simulink model "Experiments"  (R2024b)
settings: Solver=ode1  StartTime=0.0  StopTime=30  FixedStep=0.002  RelTol=1e-3  EnableMultiTasking=on
values from neighbouring files (symbols this model uses):
  A = [-2  1  -1  1  0  0 ... (first row only)    [observer_sim.m]    (also in setup_experiments.m = -19.637526957)
  B = eye(n_x,n_u)    [observer_sim.m]    (also in setup_experiments.m = 23*sqrt(4+A^2))
  C = eye(n_y,n_x)    [observer_sim.m]    (also in setup_experiments.m = 1)
  d1_max = 0.8    [observer_sim.m]    (also in setup_experiments.m)
  d1_min = 0.2    [observer_sim.m]    (also in setup_experiments.m)
  epsilon = 0.01    [observer_sim.m]    (also in setup_experiments.m = 0.05)
  L_region1_R = zeros(n_x+n_u, n_y, 2^n_u)    [observer_sim.m]    (also in setup_experiments.m)
  L_region2_R = zeros(n_x+n_u, n_y, 2^n_u)    [observer_sim.m]    (also in setup_experiments.m)
  M = 5    [setup_experiments.m]
  n_u = 2    [observer_sim.m]    (also in setup_experiments.m = 1)
  n_x = 6    [observer_sim.m]    (also in setup_experiments.m = 1)
  n_y = 2    [observer_sim.m]    (also in setup_experiments.m = 1)
  u1dot_max = 10    [observer_sim.m]    (also in setup_experiments.m = 5)
  u1dot_min = -10    [observer_sim.m]    (also in setup_experiments.m = -5)
  w = 1    [setup_experiments.m]
undefined symbols (not defined in the file or in its folder): HIL, qc_get_step_size
libraries: quarc_library x3
settings Model: SimulationMode=external  ExtModeTrigDuration=40000  Creator=MLevis  LastModifiedBy=torivarhaughom
settings SolverCC: AlgebraicLoopSolver=TrustRegion  PositivePriorityOrder=on
settings DataIOCC: SaveFormat=Array  SignalLoggingSaveFormat=ModelDataLogs  ReturnWorkspaceOutputs=off
settings OptimizationCC: ExpressionDepthLimit=2147483647  LifeSpan=inf
settings DebuggingCC: UnderspecifiedInitializationDetection=Classic  MergeDetectMultiDrivingBlocksExec=none  SolverPrmCheckMsg=warning  FcnCallInpInsideContextMsg=warning  UnconnectedInputMsg=warning  UnconnectedOutputMsg=warning  UnconnectedLineMsg=warning  StateNameClashWarn=warning  SFUnexpectedBacktrackingDiag=warning  SFNoUnconditionalDefaultTransitionDiag=warning  SFExecutionAtInitializationDiag=none  ArithmeticOperatorsInVariantConditions=warning
settings HardwareCC: ProdBitPerPointer=32  ProdBitPerSizeT=32  ProdBitPerPtrDiffT=32  ProdLargestAtomicFloat=None  ProdIntDivRoundTo=Undefined  ProdEndianess=Unspecified  ProdWordSize=32  ProdHWDeviceType=32-bit Generic
settings ModelReferenceCC: EnableRefExpFcnMdlSchedulingChecks=on  PropagateSignalLabelsOutOfModel=off
settings SFSimCC: SimUseLocalCustomCode=off  CustomCodeUndefinedFunction=UseInterfaceOnly
settings RTWCC: Description=QUARC Win64 Target  SystemTargetFile=quarc_win64.tlc  TemplateMakefile=quarc_default_tmf  RTWUseLocalCustomCode=off  GPUComputeCapability=3.5  DLArmComputeVersion=19.05
settings CodeAppCC: StateflowObjectComments=on
settings STFCustomTargetCC: TargetPreCompLibLocation=C:\PROGRA~3\QUARC\lib\2020b\win64\release  ConcurrentExecutionCompliant=on  CombineOutputUpdateFcns=on  CPPClassGenCompliant=on  SystemTargetFile=quarc_win64.tlc
settings GRTTargetCC: TargetPreCompLibLocation=C:\PROGRA~3\QUARC\lib\2020b\win64\release  TargetLangStandard=C89/C90 (ANSI)  ParMdlRefBuildCompliant=off  CompOptLevelCompliant=off  MatFileLogging=off  UseToolchainInfoCompliant=off  ExtMode=on  ExtModeMexFile=quarc_comm
settings ConfigComp: CovMetricSettings=dw  CovSaveCumulativeToWorkspaceVar=on  CovSaveSingleToWorkspaceVar=on  CovExternalEMLEnable=off  CovSFcnEnable=off

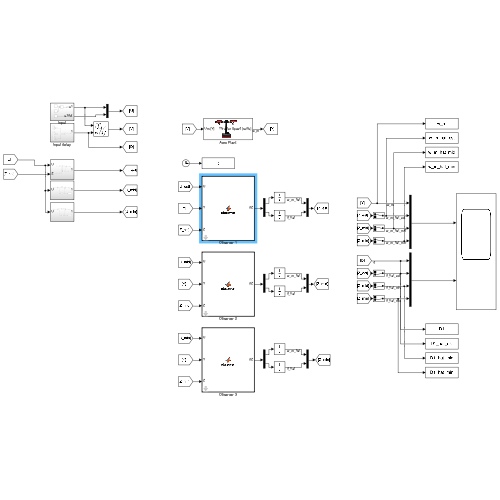
[thumbnail: Simulink's stored preview of the top-level diagram]
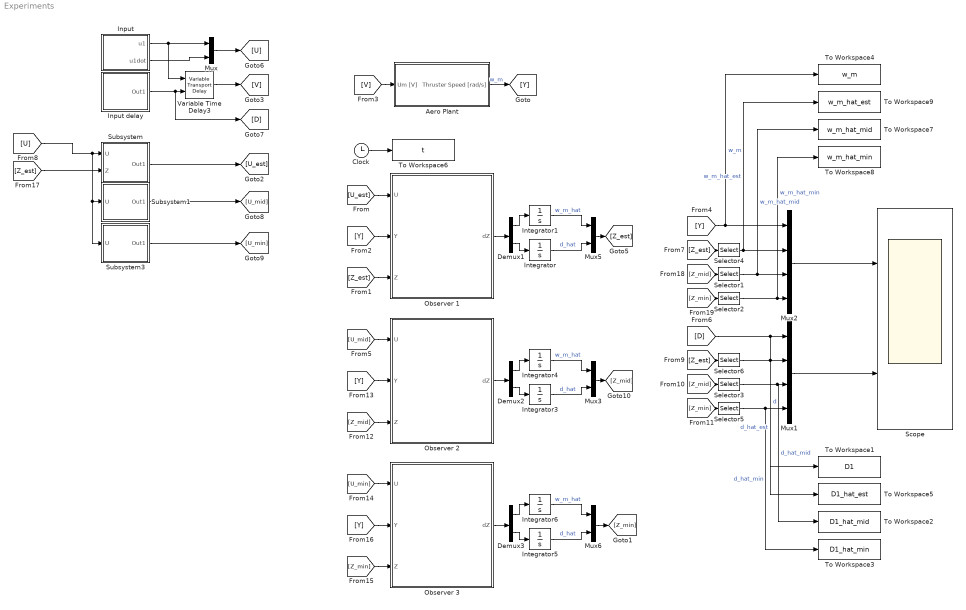
== system Experiments ==
  Aero Plant : Subsystem
      mask Display: image('$imagefile'); % Use "Edit Image" on toolstrip to change.
  Clock : Clock
  Demux1 : Demux  Outputs=2
  Demux2 : Demux  Outputs=2
  Demux3 : Demux  Outputs=2
  Input : Subsystem
  Input delay : Subsystem
  Integrator : Integrator  InitialCondition=(d1_min+d1_max)/2
  Integrator1 : Integrator
  Integrator3 : Integrator  InitialCondition=(d1_min+d1_max)/2
  Integrator4 : Integrator
  Integrator5 : Integrator  InitialCondition=(d1_min+d1_max)/2
  Integrator6 : Integrator
  Mux{,3,5..6} (4 alike) : Mux  Inputs=2
  Mux1 : Mux
  Mux2 : Mux
  Observer 1 : MATLAB Function  TreatAsAtomicUnit=on  mask{A=A, B=B, C=C, dimensions=[n_x, n_u, n_y], d_limits=[d1_min, d1_max], udot_limits=[u1dot_min, u1dot_max], epsilon=epsilon, L_region1_R=L_region1_R, L_region2_R=L_region2_R, perturbation=0}
      mask prompts: dimensions "[n_x, n_u, n_y]"; d_limits "[d_min, d_max]"; udot_limits "[udot_min, udot_max]"; perturbation "Estimate remainder term"
  Observer 2 : MATLAB Function  TreatAsAtomicUnit=on  mask{A=A, B=B, C=C, dimensions=[n_x, n_u, n_y], d_limits=[d1_min, d1_max], udot_limits=[u1dot_min, u1dot_max], epsilon=epsilon, L_region1_R=L_region1_R, L_region2_R=L_region2_R, perturbation=0}
      mask prompts: dimensions "[n_x, n_u, n_y]"; d_limits "[d_min, d_max]"; udot_limits "[udot_min, udot_max]"; perturbation "Estimate remainder term"
  Observer 3 : MATLAB Function  TreatAsAtomicUnit=on  mask{A=A, B=B, C=C, dimensions=[n_x, n_u, n_y], d_limits=[d1_min, d1_max], udot_limits=[u1dot_min, u1dot_max], epsilon=epsilon, L_region1_R=L_region1_R, L_region2_R=L_region2_R, perturbation=0}
      mask prompts: dimensions "[n_x, n_u, n_y]"; d_limits "[d_min, d_max]"; udot_limits "[udot_min, udot_max]"; perturbation "Estimate remainder term"
  Scope : Scope  NumInputPorts=2
  Selector1 : Selector  InputPortWidth=2  IndexOptions=Index vector (dialog)  Indices=1  OutputSizes=1
  Selector2 : Selector  InputPortWidth=2  IndexOptions=Index vector (dialog)  Indices=1  OutputSizes=1
  Selector3 : Selector  InputPortWidth=2  IndexOptions=Index vector (dialog)  Indices=2  OutputSizes=1
  Selector4 : Selector  InputPortWidth=2  IndexOptions=Index vector (dialog)  Indices=1  OutputSizes=1
  Selector5 : Selector  InputPortWidth=2  IndexOptions=Index vector (dialog)  Indices=2  OutputSizes=1
  Selector6 : Selector  InputPortWidth=2  IndexOptions=Index vector (dialog)  Indices=2  OutputSizes=1
  Subsystem : Subsystem
  Subsystem1 : Subsystem
  Subsystem3 : Subsystem
  To Workspace1 : ToWorkspace  VariableName=D1  SampleTime=-1
  To Workspace2 : ToWorkspace  VariableName=D1_hat_mid  SampleTime=-1
  To Workspace3 : ToWorkspace  VariableName=D1_hat_min  SampleTime=-1
  To Workspace4 : ToWorkspace  VariableName=w_m  SampleTime=-1
  To Workspace5 : ToWorkspace  VariableName=D1_hat_est  SampleTime=-1
  To Workspace6 : ToWorkspace  VariableName=t  SampleTime=-1
  To Workspace7 : ToWorkspace  VariableName=w_m_hat_mid  SampleTime=-1
  To Workspace8 : ToWorkspace  VariableName=w_m_hat_min  SampleTime=-1
  To Workspace9 : ToWorkspace  VariableName=w_m_hat_est  SampleTime=-1
  Variable Time Delay3 : VariableTransportDelay  MaximumDelay=10  MaximumPoints=10240
  wires:
  Integrator/1 -> Mux5/2  "d_hat"
  Integrator1/1 -> Mux5/1  "w_m_hat"
  Demux1/2 -> Integrator/1
  Demux1/1 -> Integrator1/1
  Aero Plant/1(Thruster Speed [rad/s]) -> [Y]  "w_m"
  Observer 1/1(dZ) -> Demux1/1
  [Z_est] -> Observer 1/3(Z)
  [U_est] -> Observer 1/1(U)
  [Y] -> Observer 1/2(Y)
  Mux5/1 -> [Z_est]
  [V] -> Aero Plant/1(Um [V])
  Variable Time Delay3/1 -> [V]
  Input/1(u1) -> Mux/1, Variable Time Delay3/1
  Input delay/1(Out1) -> [D], Variable Time Delay3/2
  [U_mid] -> Observer 2/1(U)
  [Y] -> Observer 2/2(Y)
  Observer 2/1(dZ) -> Demux2/1
  Integrator3/1 -> Mux3/2  "d_hat"
  [Z_mid] -> Observer 2/3(Z)
  Mux3/1 -> [Z_mid]
  Demux2/2 -> Integrator3/1
  Integrator4/1 -> Mux3/1  "w_m_hat"
  Demux2/1 -> Integrator4/1
  [U_min] -> Observer 3/1(U)
  [Y] -> Observer 3/2(Y)
  Observer 3/1(dZ) -> Demux3/1
  Integrator5/1 -> Mux6/2  "d_hat"
  [Z_min] -> Observer 3/3(Z)
  Mux6/1 -> [Z_min]
  Demux3/2 -> Integrator5/1
  Integrator6/1 -> Mux6/1  "w_m_hat"
  Demux3/1 -> Integrator6/1
  Mux/1 -> [U]
  Input/2(u1dot) -> Mux/2
  Subsystem/1(Out1) -> [U_est]
  Subsystem1/1(Out1) -> [U_mid]
  Subsystem3/1(Out1) -> [U_min]
  Clock/1 -> To Workspace6/1
  Selector5/1 -> To Workspace3/1, Mux1/4  "d_hat_min"
  Mux2/1 -> Scope/1
  Selector2/1 -> To Workspace8/1, Mux2/4  "w_m_hat_min"
  [Z_min] -> Selector2/1
  [Z_est] -> Selector6/1
  [Z_min] -> Selector5/1
  Selector1/1 -> Mux2/3, To Workspace7/1  "w_m_hat_mid"
  [Z_est] -> Selector4/1
  Selector3/1 -> To Workspace2/1, Mux1/3  "d_hat_mid"
  [Z_mid] -> Selector3/1
  Selector6/1 -> To Workspace5/1, Mux1/2  "d_hat_est"
  [Y] -> Mux2/1, To Workspace4/1  "w_m"
  Mux1/1 -> Scope/2
  [Z_mid] -> Selector1/1
  Selector4/1 -> Mux2/2, To Workspace9/1  "w_m_hat_est"
  [D] -> Mux1/1, To Workspace1/1  "d"
  [U] -> Subsystem3/1(U), Subsystem1/1(U), Subsystem/1(U)
  [Z_est] -> Subsystem/2(Z)

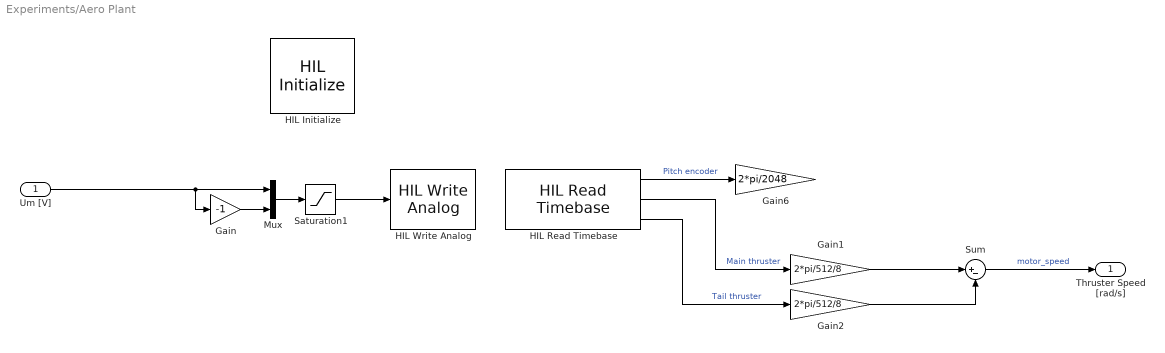
== system Experiments/Aero Plant ==
  Um [V] : Inport
  Gain : Gain  Gain=-1
  Gain1 : Gain  Gain=2*pi/512/8
  Gain2 : Gain  Gain=2*pi/512/8
  Gain6 : Gain  Gain=2*pi/2048
  HIL Initialize : quarc_library/Data Acquisition/Generic/Configuration/HIL Initialize  Priority=-99  object_name=HIL-1  board_type=---- Quanser ----  board_number=0  board_options=""  exclusive=off  active=off  hardware_clocks=[0]  clock_modes=[]  initial_clock_frequencies=[]  set_clock_params_at_start=off  set_clock_params_at_switch_in=off  set_clock_frequencies_at_start=off  set_clock_frequencies_at_switch_in=off  analog_input_channels=[0:1]  analog_input_configurations=[]  analog_input_maximums=3  analog_input_minimums=-3  set_analog_input_params_at_start=off  set_analog_input_params_at_switch_in=off  analog_output_channels=[0:1]  analog_output_maximums=24  analog_output_minimums=-24  initial_analog_outputs=[0]  final_analog_outputs=[0]  watchdog_analog_outputs=[0]  set_analog_output_params_at_start=off  set_analog_output_params_at_switch_in=off  set_analog_outputs_at_start=on  set_analog_outputs_at_switch_in=off  set_analog_outputs_at_terminate=on  set_analog_outputs_at_switch_out=off  set_analog_outputs_on_watchdog=off  digital_input_channels=[]  digital_output_channels=[0:1]  digital_output_configuration=[]  initial_digital_outputs=[1]  final_digital_outputs=[0]  watchdog_digital_outputs=[0]  set_digital_output_params_at_start=off  set_digital_output_params_at_switch_in=off  set_digital_outputs_at_start=on  set_digital_outputs_at_switch_in=off  set_digital_outputs_at_terminate=on  set_digital_outputs_at_switch_out=off  set_digital_outputs_on_watchdog=off  encoder_channels=[0:3]  quadrature=[4]  encoder_filter_frequency=[]  initial_encoder_counts=[0]  set_encoder_params_at_start=off  set_encoder_params_at_switch_in=off  set_encoder_counts_at_start=on  set_encoder_counts_at_switch_in=off  pwm_channels=[]  pwm_modes=[]  pwm_frequency=[]  pwm_configuration=[]  pwm_alignment=[]  pwm_polarity=[]  pwm_leading_deadband=[]  pwm_trailing_deadband=[]  initial_pwm_outputs=[]  final_pwm_outputs=[]  watchdog_pwm_outputs=[]  set_pwm_params_at_start=off  set_pwm_params_at_switch_in=off  set_pwm_outputs_at_start=off  set_pwm_outputs_at_switch_in=off  set_pwm_outputs_at_terminate=off  set_pwm_outputs_at_switch_out=off  set_pwm_outputs_on_watchdog=off  other_output_channels=[11000:11002]  initial_other_outputs=[0 1 0]  final_other_outputs=[1 0 0]  watchdog_other_outputs=[0 0 1]  set_other_outputs_at_start=on  set_other_outputs_at_switch_in=off  set_other_outputs_at_terminate=on  set_other_outputs_at_switch_out=off  set_other_outputs_on_watchdog=off
  HIL Read Timebase : quarc_library/Data Acquisition/Generic/Timebases/HIL Read Timebase  object_name=HIL-1  clock=0  analog_channels=[]  encoder_channels=[2]  digital_channels=[]  other_channels=[14000 14001]  active=on  vector_output=off  data_type_mode=Inherit via back propagation  encoder_data_type=double  digital_data_type=boolean  overflow_mode=Error on overflow  samples_in_buffer=max(ceil(1/qc_get_step_size), 1)
  HIL Write Analog : quarc_library/Data Acquisition/Generic/Immediate I//O/HIL Write Analog  object_name=HIL-1  channels=[0:1]  sample_time=-1  active=off  vector_input=on
  Mux : Mux  Inputs=2
  Saturation1 : Saturate  UpperLimit=24  LowerLimit=-24
  Sum : Sum  Inputs=|+-
  Thruster Speed [rad/s] : Outport
  wires:
  Mux/1 -> Saturation1/1
  Gain/1 -> Mux/2
  Um [V]/1 -> Gain/1, Mux/1
  Gain2/1 -> Sum/2
  Sum/1 -> Thruster Speed [rad/s]/1  "motor_speed"
  HIL Read Timebase/2 -> Gain1/1  "Main thruster"
  HIL Read Timebase/3 -> Gain2/1  "Tail thruster"
  HIL Read Timebase/1 -> Gain6/1  "Pitch encoder"
  Gain1/1 -> Sum/1
  Saturation1/1 -> HIL Write Analog/1

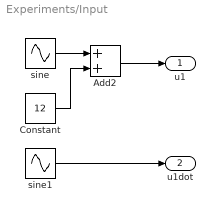
== system Experiments/Input ==
  Add2 : Sum
  Constant : Constant  Value=12
  sine : Sin  Amplitude=M  Frequency=w  SampleTime=0
  sine1 : Sin  Amplitude=M*w  Frequency=w  Phase=pi/2  SampleTime=0
  u1 : Outport
  u1dot : Outport  Port=2
  wires:
  Constant/1 -> Add2/2
  sine/1 -> Add2/1
  Add2/1 -> u1/1
  sine1/1 -> u1dot/1

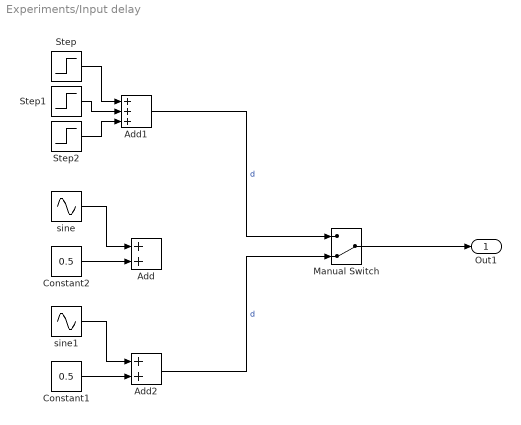
== system Experiments/Input delay ==
  Add : Sum
  Add1 : Sum  Inputs=+++
  Add2 : Sum
  Constant1 : Constant  Value=0.5
  Constant2 : Constant  Value=0.5
  Manual Switch : ManualSwitch  CurrentSetting=0
  Step : Step  Time=0  After=0.3  SampleTime=0
  Step1 : Step  Time=10  After=0.4  SampleTime=0
  Step2 : Step  Time=20  After=-0.2  SampleTime=0
  sine : Sin  Amplitude=0.3  Frequency=0.4  SampleTime=0
  sine1 : Sin  Amplitude=0.3  SampleTime=0
  Out1 : Outport
  wires:
  Constant2/1 -> Add/2
  Step2/1 -> Add1/3
  sine/1 -> Add/1
  Step/1 -> Add1/1
  Step1/1 -> Add1/2
  Manual Switch/1 -> Out1/1
  Add1/1 -> Manual Switch/1  "d"
  sine1/1 -> Add2/1
  Constant1/1 -> Add2/2
  Add2/1 -> Manual Switch/2  "d"

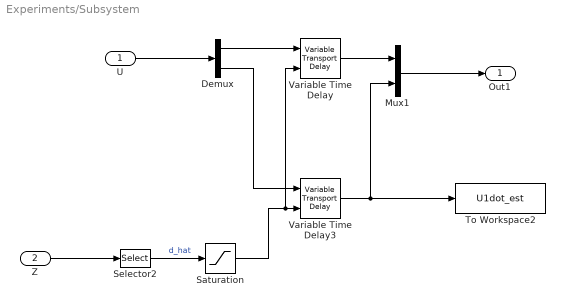
== system Experiments/Subsystem ==
  U : Inport
  Z : Inport  Port=2
  Demux : Demux  Outputs=2
  Mux1 : Mux  Inputs=2
  Saturation : Saturate  UpperLimit=d1_max  LowerLimit=d1_min
  Selector2 : Selector  InputPortWidth=2  IndexOptions=Index vector (dialog)  Indices=2  OutputSizes=1
  To Workspace2 : ToWorkspace  VariableName=U1dot_est  SampleTime=-1
  Variable Time Delay : VariableTransportDelay  MaximumDelay=10
  Variable Time Delay3 : VariableTransportDelay  MaximumDelay=10
  Out1 : Outport
  wires:
  Variable Time Delay/1 -> Mux1/1
  Mux1/1 -> Out1/1
  Variable Time Delay3/1 -> To Workspace2/1, Mux1/2
  Demux/1 -> Variable Time Delay/1
  Demux/2 -> Variable Time Delay3/1
  U/1 -> Demux/1
  Z/1 -> Selector2/1
  Selector2/1 -> Saturation/1  "d_hat"
  Saturation/1 -> Variable Time Delay/2, Variable Time Delay3/2

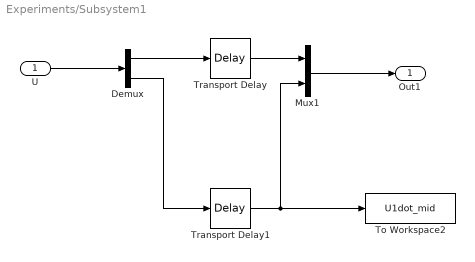
== system Experiments/Subsystem1 ==
  U : Inport
  Demux : Demux  Outputs=2
  Mux1 : Mux  Inputs=2
  To Workspace2 : ToWorkspace  VariableName=U1dot_mid  SampleTime=-1
  Transport Delay : TransportDelay  DelayTime=(d1_min+d1_max)/2
  Transport Delay1 : TransportDelay  DelayTime=(d1_min+d1_max)/2
  Out1 : Outport
  wires:
  Transport Delay/1 -> Mux1/1
  Mux1/1 -> Out1/1
  Transport Delay1/1 -> To Workspace2/1, Mux1/2
  Demux/1 -> Transport Delay/1
  Demux/2 -> Transport Delay1/1
  U/1 -> Demux/1

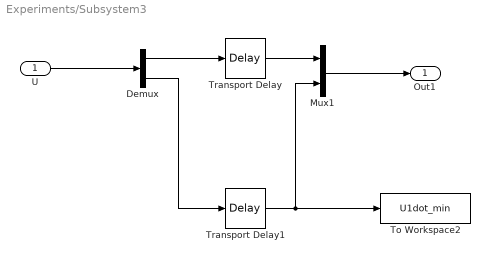
== system Experiments/Subsystem3 ==
  U : Inport
  Demux : Demux  Outputs=2
  Mux1 : Mux  Inputs=2
  To Workspace2 : ToWorkspace  VariableName=U1dot_min  SampleTime=-1
  Transport Delay : TransportDelay  DelayTime=d1_min
  Transport Delay1 : TransportDelay  DelayTime=d1_min
  Out1 : Outport
  wires:
  Transport Delay/1 -> Mux1/1
  Mux1/1 -> Out1/1
  Transport Delay1/1 -> To Workspace2/1, Mux1/2
  Demux/1 -> Transport Delay/1
  Demux/2 -> Transport Delay1/1
  U/1 -> Demux/1

== matlab function Experiments/Observer 2 ==
  settings: updateMethod=DISCRETE
  data: U input; Y input; dZ output; Z input; A parameter; B parameter; C parameter; dimensions parameter; d_limits parameter; udot_limits parameter; epsilon parameter; L_region1_R parameter; L_region2_R parameter
function dZ = observer(U, Y, Z, A, B, C, dimensions, d_limits, udot_limits, ...
                       epsilon, L_region1_R, L_region2_R)
persistent considered_region

% Define system dimensions
n_x = dimensions(1);
n_u = dimensions(2);
n_y = dimensions(3);

% Define delay and input derivative bounds
d1_min = d_limits(1); d1_max = d_limits(2); d1_mid = (d1_min+d1_max)/2;
u1dot_min = udot_limits(1); u1dot_max = udot_limits(2);

% Use mid-point value
d1_star = d1_mid;

% Inputs for augmented system
u1_ = U(1);
u1dot_ = U(2);

% Determine active region
if isempty(considered_region)
    % Initial region
    if(u1dot_ >= 0)
        considered_region = 1;
    else
        considered_region = 2;
    end
else
    if(considered_region == 1)
        if(u1dot_ < -epsilon)
            considered_region = 2;
        else
            considered_region = 1;
        end
    elseif(considered_region == 2)
        if(u1dot_ > epsilon)
            considered_region = 1;
        else
            considered_region = 2;
        end
    end
end

% Compute observer gain by bilinear interpolation based on active region
k = 1; L0 = zeros(n_x+n_u,n_y);
L_region1 = L_region1_R;
L_region2 = L_region2_R;
if(considered_region == 1)
    for temp_udot1 = [(u1dot_max-u1dot_)/(u1dot_max-(-epsilon)) (u1dot_-(-epsilon))/(u1dot_max-(-epsilon))]
            L0 = L0+temp_udot1*L_region1(:,:,k);
            k = k+1;
    end
elseif(considered_region == 2)
    for temp_udot1 = [(epsilon-u1dot_)/(epsilon-u1dot_min) (u1dot_-u1dot_min)/(epsilon-u1dot_min)]
            L0 = L0+temp_udot1*L_region2(:,:,k);
            k = k+1;
    end
end

% Construct augmented system matrices for the observer
U_dot = u1dot_; 
D_ = d1_star;

A_ = [A  -B*U_dot ;
     zeros(n_u,n_x) zeros(n_u,n_u)];
B_ = [B B*D_ ;
      zeros(n_u,n_u) zeros(n_u,n_u)];
C_ = [C zeros(n_y,n_u)];

% Z(1):   estimate of the state
% Z(2):   estimate of the delay
dZ = zeros(2,1);

% Dynamics of the observer
dZ(1:2) = A_*Z(1:2)+B_*[u1_ ; u1dot_]...
    -L0*(C_*Z(1:2)-Y);

== matlab function Experiments/Observer 1 ==
  settings: updateMethod=DISCRETE
  data: U input; Y input; dZ output; Z input; A parameter; B parameter; C parameter; dimensions parameter; d_limits parameter; udot_limits parameter; epsilon parameter; L_region1_R parameter; L_region2_R parameter
function dZ = observer(U, Y, Z, A, B, C, dimensions, d_limits, udot_limits, ...
                       epsilon, L_region1_R, L_region2_R)
persistent considered_region

% Define system dimensions
n_x = dimensions(1);
n_u = dimensions(2);
n_y = dimensions(3);

% Define delay and input derivative bounds
d1_min = d_limits(1); d1_max = d_limits(2);
u1dot_min = udot_limits(1); u1dot_max = udot_limits(2);

% Use saturated delay estimates
d1_hat_sat = Z(2);
if d1_hat_sat > d1_max
    d1_hat_sat = d1_max;
elseif d1_hat_sat < d1_min
    d1_hat_sat = d1_min;
end
d1_star = d1_hat_sat;


% Inputs for augmented system
u1_ = U(1);
u1dot_ = U(2);

% Determine active region
if isempty(considered_region)
    % Initial region
    if(u1dot_ >= 0)
        considered_region = 1;
    else
        considered_region = 2;
    end
else
    if(considered_region == 1)
        if(u1dot_ < -epsilon)
            considered_region = 2;
        else
            considered_region = 1;
        end
    elseif(considered_region == 2)
        if(u1dot_ > epsilon)
            considered_region = 1;
        else
            considered_region = 2;
        end
    end
end

% Compute observer gain by bilinear interpolation based on active region
k = 1; 
L0 = zeros(n_x+n_u,n_y);
L_region1 = L_region1_R;
L_region2 = L_region2_R;
if(considered_region == 1)
    for temp_udot1 = [(u1dot_max-u1dot_)/(u1dot_max-(-epsilon)) (u1dot_-(-epsilon))/(u1dot_max-(-epsilon))]
            L0 = L0+temp_udot1*L_region1(:,:,k);
            k = k+1;
    end
elseif(considered_region == 2)
    for temp_udot1 = [(epsilon-u1dot_)/(epsilon-u1dot_min) (u1dot_-u1dot_min)/(epsilon-u1dot_min)]
            L0 = L0+temp_udot1*L_region2(:,:,k);
            k = k+1;
    end
end

% Construct augmented system matrices for the observer
U_dot = u1dot_; 
D_ = d1_star;

A_ = [A  -B*U_dot ;
     zeros(n_u,n_x) zeros(n_u,n_u)];
B_ = [B B*D_ ;
      zeros(n_u,n_u) zeros(n_u,n_u)];
C_ = [C zeros(n_y,n_u)];

% Z(1):   estimate of the state
% Z(2):   estimate of the delay
dZ = zeros(2,1);

% Dynamics of the observer
dZ(1:2) = A_*Z(1:2)+B_*[u1_ ; u1dot_]...
    -L0*(C_*Z(1:2)-Y);

== matlab function Experiments/Observer 3 ==
  settings: updateMethod=DISCRETE
  data: U input; Y input; dZ output; Z input; A parameter; B parameter; C parameter; dimensions parameter; d_limits parameter; udot_limits parameter; epsilon parameter; L_region1_R parameter; L_region2_R parameter
function dZ = observer(U, Y, Z, A, B, C, dimensions, d_limits, udot_limits, ...
                       epsilon, L_region1_R, L_region2_R)
persistent considered_region

% Define system dimensions
n_x = dimensions(1);
n_u = dimensions(2);
n_y = dimensions(3);

% Define delay and input derivative bounds
d1_min = d_limits(1); d1_max = d_limits(2);
u1dot_min = udot_limits(1); u1dot_max = udot_limits(2);

% Use lower bound
d1_star = d1_min;

% Inputs for augmented system
u1_ = U(1);
u1dot_ = U(2);

% Determine active region
if isempty(considered_region)
    % Initial region
    if(u1dot_ >= 0)
        considered_region = 1;
    else
        considered_region = 2;
    end
else
    if(considered_region == 1)
        if(u1dot_ < -epsilon)
            considered_region = 2;
        else
            considered_region = 1;
        end
    elseif(considered_region == 2)
        if(u1dot_ > epsilon)
            considered_region = 1;
        else
            considered_region = 2;
        end
    end
end

% Compute observer gain by bilinear interpolation based on active region
k = 1; L0 = zeros(n_x+n_u,n_y);
L_region1 = L_region1_R;
L_region2 = L_region2_R;
if(considered_region == 1)
    for temp_udot1 = [(u1dot_max-u1dot_)/(u1dot_max-(-epsilon)) (u1dot_-(-epsilon))/(u1dot_max-(-epsilon))]
            L0 = L0+temp_udot1*L_region1(:,:,k);
            k = k+1;
    end
elseif(considered_region == 2)
    for temp_udot1 = [(epsilon-u1dot_)/(epsilon-u1dot_min) (u1dot_-u1dot_min)/(epsilon-u1dot_min)]
            L0 = L0+temp_udot1*L_region2(:,:,k);
            k = k+1;
    end
end

% Construct augmented system matrices for the observer
U_dot = u1dot_; 
D_ = d1_star;

A_ = [A  -B*U_dot ;
     zeros(n_u,n_x) zeros(n_u,n_u)];
B_ = [B B*D_ ;
      zeros(n_u,n_u) zeros(n_u,n_u)];
C_ = [C zeros(n_y,n_u)];

% Z(1):   estimate of the state
% Z(2):   estimate of the delay
dZ = zeros(2,1);

% Dynamics of the observer
dZ(1:2) = A_*Z(1:2)+B_*[u1_ ; u1dot_]...
    -L0*(C_*Z(1:2)-Y);
